simulink subsystem "Control_Selector"  (R2025a)
settings: Solver=VariableStepAuto  StartTime=0.0  StopTime=10.0  RelTol=1e-3
settings Model: Creator=gurt1  LastModifiedBy=gurt1

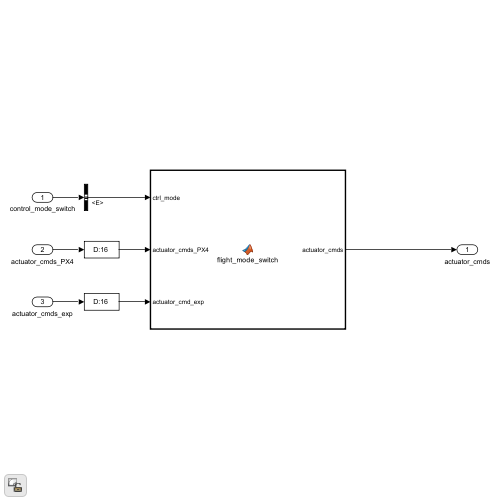
[thumbnail: Simulink's stored preview of the top-level diagram]
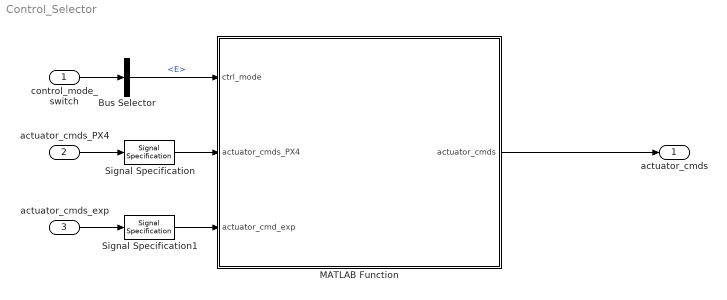
== system Control_Selector ==
  control_mode_switch : Inport
  actuator_cmds_PX4 : Inport  Port=2
  actuator_cmds_exp : Inport  Port=3
  Bus Selector : BusSelector  OutputSignals=switches.E
  MATLAB Function : MATLAB Function  TreatAsAtomicUnit=on
  Signal Specification : SignalSpecification  Dimensions=16
  Signal Specification1 : SignalSpecification  Dimensions=16
  actuator_cmds : Outport
  wires:
  actuator_cmds_PX4/1 -> Signal Specification/1
  actuator_cmds_exp/1 -> Signal Specification1/1
  MATLAB Function/1(actuator_cmds) -> actuator_cmds/1
  Bus Selector/1 -> MATLAB Function/1(ctrl_mode)  "<E>"
  Signal Specification/1 -> MATLAB Function/2(actuator_cmds_PX4)
  Signal Specification1/1 -> MATLAB Function/3(actuator_cmd_exp)
  control_mode_switch/1 -> Bus Selector/1

== matlab function Control_Selector/MATLAB Function ==
  data: ctrl_mode input; actuator_cmds output; actuator_cmds_PX4 input; actuator_cmd_exp input
function actuator_cmds = flight_mode_switch(ctrl_mode, actuator_cmds_PX4, actuator_cmd_exp)

if ctrl_mode > 0.5
    actuator_cmds = actuator_cmds_PX4;
else
    actuator_cmds = actuator_cmd_exp;
end
